simulink model "power_law_adapter"  (R2020b)
settings: Solver=FixedStepDiscrete  StartTime=0.0  StopTime=stopTime  FixedStep=2.0833333333333333e-05  RelTol=1e-3
undefined symbols (not defined in the file or in its folder): alpha1, alpha2, fast_coeffs, slow_coeffs
settings Model: Creator=Ross  LastModifiedBy=tyler
settings DataIOCC: SaveOutput=off  SaveTime=off  ReturnWorkspaceOutputs=off
settings OptimizationCC: BlockReduction=off  ConditionallyExecuteInputs=off  DefaultParameterBehavior=Inlined
settings DebuggingCC: ReadBeforeWriteMsg=DisableAll  WriteAfterWriteMsg=DisableAll  WriteAfterReadMsg=DisableAll  AlgebraicLoopMsg=error  MultiTaskDSMMsg=none  SingleTaskRateTransMsg=error  PregeneratedLibrarySubsystemCodeDiagnostic=none  ArithmeticOperatorsInVariantConditions=warning
settings HardwareCC: ProdBitPerPointer=32  ProdBitPerSizeT=32  ProdBitPerPtrDiffT=32  ProdLargestAtomicFloat=None  ProdIntDivRoundTo=Undefined  ProdEndianess=Unspecified  ProdWordSize=32  ProdHWDeviceType=ASIC/FPGA->ASIC/FPGA  TargetBitPerPointer=64  TargetBitPerSizeT=64  TargetBitPerPtrDiffT=64  TargetLongLongMode=on  TargetIntDivRoundTo=Zero  TargetEndianess=LittleEndian  TargetWordSize=64  TargetHWDeviceType=Custom Processor->MATLAB Host Computer  ProdEqTarget=off
settings ModelReferenceCC: UpdateModelReferenceTargets=IfOutOfDate
settings SFSimCC: SFSimEcho=off  SimUseLocalCustomCode=off  CustomCodeUndefinedFunction=UseInterfaceOnly
settings RTWCC: RTWUseLocalCustomCode=off

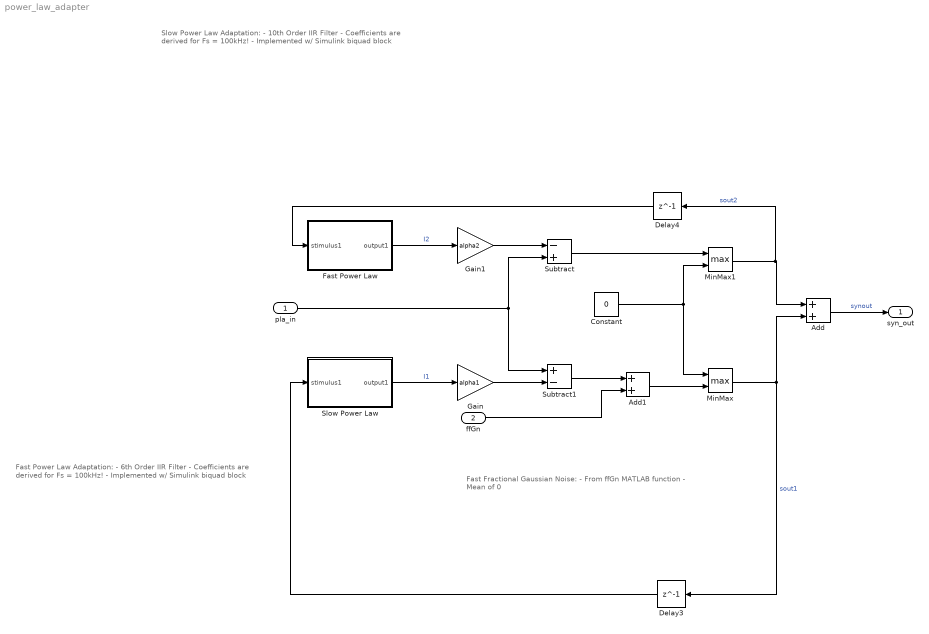
== system power_law_adapter ==
  note: Slow Power Law Adaptation:
      |
      | - 10th Order IIR Filter
      |
      | - Coefficients are derived for Fs = 100kHz!
      |
      | - Implemented w/ Simulink biquad block
  note: Fast Power Law Adaptation:
      |
      | - 6th Order IIR Filter
      |
      | - Coefficients are derived for Fs = 100kHz!
      |
      | - Implemented w/ Simulink biquad block
  note: Fast Fractional Gaussian Noise:
      |
      | - From ffGn MATLAB function
      |
      | - Mean of 0
  pla_in : Inport  OutDataTypeStr=single  PortDimensions=1  SampleTime=[2.0833333333333333e-05,0]
  ffGn : Inport  Port=2  OutDataTypeStr=single  PortDimensions=[1 1]  SampleTime=[2.0833333333333333e-05,0]
  Add : Sum
  Add1 : Sum
  Constant : Constant  Value=0  OutDataTypeStr=single  SampleTime=-1
  Delay3 : Delay  DelayLength=1
  Delay4 : Delay  DelayLength=1
  Fast Power Law : Subsystem
  Gain : Gain  Gain=alpha1  ParamDataTypeStr=single  OutDataTypeStr=single
  Gain1 : Gain  Gain=alpha2  ParamDataTypeStr=single  OutDataTypeStr=single
  MinMax : MinMax  Function=max  Inputs=2
  MinMax1 : MinMax  Function=max  Inputs=2
  Slow Power Law : Subsystem
  Subtract : Sum  Inputs=-+
  Subtract1 : Sum  Inputs=+-
  syn_out : Outport  OutDataTypeStr=single  PortDimensions=1  SampleTime=[2.0833333333333333e-05,0]
  wires:
  Subtract/1 -> MinMax1/1
  MinMax1/1 -> Delay4/1, Add/1  "sout2"
  Gain/1 -> Subtract1/2
  Fast Power Law/1(output1) -> Gain1/1  "I2"
  Gain1/1 -> Subtract/1
  Add1/1 -> MinMax/2
  Add/1 -> syn_out/1  "synout"
  Subtract1/1 -> Add1/1
  Constant/1 -> MinMax/1, MinMax1/2
  Slow Power Law/1(output1) -> Gain/1  "I1"
  MinMax/1 -> Delay3/1, Add/2  "sout1"
  Delay3/1 -> Slow Power Law/1(stimulus1)
  Delay4/1 -> Fast Power Law/1(stimulus1)
  ffGn/1 -> Add1/2
  pla_in/1 -> Subtract1/1, Subtract/2

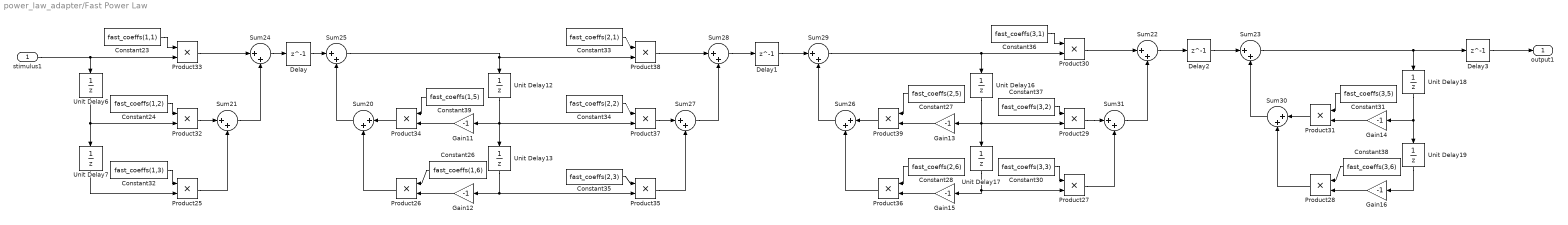
== system power_law_adapter/Fast Power Law ==
  stimulus1 : Inport
  Constant23 : Constant  Value=fast_coeffs(1,1)  OutDataTypeStr=single  SampleTime=-1
  Constant24 : Constant  Value=fast_coeffs(1,2)  OutDataTypeStr=single  SampleTime=-1
  Constant26 : Constant  Value=fast_coeffs(1,6)  OutDataTypeStr=single  SampleTime=-1
  Constant27 : Constant  Value=fast_coeffs(2,5)  OutDataTypeStr=single  SampleTime=-1
  Constant28 : Constant  Value=fast_coeffs(2,6)  OutDataTypeStr=single  SampleTime=-1
  Constant30 : Constant  Value=fast_coeffs(3,3)  OutDataTypeStr=single  SampleTime=-1
  Constant31 : Constant  Value=fast_coeffs(3,5)  OutDataTypeStr=single  SampleTime=-1
  Constant32 : Constant  Value=fast_coeffs(1,3)  OutDataTypeStr=single  SampleTime=-1
  Constant33 : Constant  Value=fast_coeffs(2,1)  OutDataTypeStr=single  SampleTime=-1
  Constant34 : Constant  Value=fast_coeffs(2,2)  OutDataTypeStr=single  SampleTime=-1
  Constant35 : Constant  Value=fast_coeffs(2,3)  OutDataTypeStr=single  SampleTime=-1
  Constant36 : Constant  Value=fast_coeffs(3,1)  OutDataTypeStr=single  SampleTime=-1
  Constant37 : Constant  Value=fast_coeffs(3,2)  OutDataTypeStr=single  SampleTime=-1
  Constant38 : Constant  Value=fast_coeffs(3,6)  OutDataTypeStr=single  SampleTime=-1
  Constant39 : Constant  Value=fast_coeffs(1,5)  OutDataTypeStr=single  SampleTime=-1
  Delay{,1..3} (4 alike) : Delay  DelayLength=1
  Gain{11..16} (6 alike) : Gain  Gain=-1
  Product{25..39} (15 alike) : Product
  Sum{20..31} (12 alike) : Sum  Inputs=|++
  Unit Delay{6..7,12..13,16..19} (8 alike) : UnitDelay  SampleTime=-1  HasFrameUpgradeWarning=on
  output1 : Outport  VectorParamsAs1DForOutWhenUnconnected=off
  wires:
  Product28/1 -> Sum30/2
  Gain12/1 -> Product26/2
  Constant28/1 -> Product36/1
  Constant31/1 -> Product31/1
  Constant38/1 -> Product28/1
  Constant37/1 -> Product29/1
  Constant30/1 -> Product27/1
  Product29/1 -> Sum31/1
  Unit Delay18/1 -> Unit Delay19/1, Gain14/1
  Constant36/1 -> Product30/1
  Sum31/1 -> Sum22/2
  Gain14/1 -> Product31/2
  Product35/1 -> Sum27/2
  Constant24/1 -> Product32/1
  Product36/1 -> Sum26/2
  Product39/1 -> Sum26/1
  Sum30/1 -> Sum23/2
  Constant35/1 -> Product35/1
  Product25/1 -> Sum21/2
  Constant23/1 -> Product33/1
  Product30/1 -> Sum22/1
  Unit Delay13/1 -> Product35/2, Gain12/1
  Constant33/1 -> Product38/1
  Unit Delay7/1 -> Product25/2
  Unit Delay17/1 -> Product27/2, Gain15/1
  Sum29/1 -> Product30/2, Unit Delay16/1
  Sum20/1 -> Sum25/2
  Sum26/1 -> Sum29/2
  Constant27/1 -> Product39/1
  Gain16/1 -> Product28/2
  Gain15/1 -> Product36/2
  Product32/1 -> Sum21/1
  Product31/1 -> Sum30/1
  Gain13/1 -> Product39/2
  Sum27/1 -> Sum28/2
  Constant34/1 -> Product37/1
  Product33/1 -> Sum24/1
  Product27/1 -> Sum31/2
  Unit Delay12/1 -> Product37/2, Unit Delay13/1, Gain11/1
  Sum25/1 -> Product38/2, Unit Delay12/1
  Unit Delay19/1 -> Gain16/1
  Product34/1 -> Sum20/1
  Gain11/1 -> Product34/2
  Sum24/1 -> Delay/1
  Constant32/1 -> Product25/1
  Product38/1 -> Sum28/1
  Product37/1 -> Sum27/1
  Sum21/1 -> Sum24/2
  Constant39/1 -> Product34/1
  Unit Delay6/1 -> Unit Delay7/1, Product32/2
  Unit Delay16/1 -> Product29/2, Unit Delay17/1, Gain13/1
  Constant26/1 -> Product26/1
  Product26/1 -> Sum20/2
  stimulus1/1 -> Product33/2, Unit Delay6/1
  Sum23/1 -> Delay3/1, Unit Delay18/1
  Delay/1 -> Sum25/1
  Sum28/1 -> Delay1/1
  Delay1/1 -> Sum29/1
  Delay2/1 -> Sum23/1
  Sum22/1 -> Delay2/1
  Delay3/1 -> output1/1

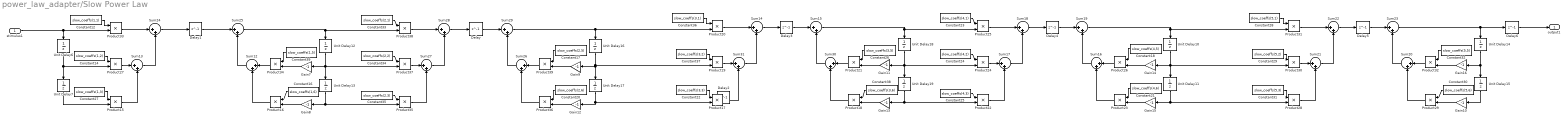
== system power_law_adapter/Slow Power Law ==
  stimulus1 : Inport
  Constant12 : Constant  Value=slow_coeffs(1,1)  OutDataTypeStr=single  SampleTime=-1
  Constant14 : Constant  Value=slow_coeffs(1,2)  OutDataTypeStr=single  SampleTime=-1
  Constant16 : Constant  Value=slow_coeffs(1,6)  OutDataTypeStr=single  SampleTime=-1
  Constant17 : Constant  Value=slow_coeffs(2,5)  OutDataTypeStr=single  SampleTime=-1
  Constant18 : Constant  Value=slow_coeffs(4,5)  OutDataTypeStr=single  SampleTime=-1
  Constant20 : Constant  Value=slow_coeffs(2,6)  OutDataTypeStr=single  SampleTime=-1
  Constant21 : Constant  Value=slow_coeffs(4,6)  OutDataTypeStr=single  SampleTime=-1
  Constant22 : Constant  Value=slow_coeffs(3,3)  OutDataTypeStr=single  SampleTime=-1
  Constant23 : Constant  Value=slow_coeffs(4,1)  OutDataTypeStr=single  SampleTime=-1
  Constant24 : Constant  Value=slow_coeffs(4,2)  OutDataTypeStr=single  SampleTime=-1
  Constant25 : Constant  Value=slow_coeffs(4,3)  OutDataTypeStr=single  SampleTime=-1
  Constant26 : Constant  Value=slow_coeffs(3,5)  OutDataTypeStr=single  SampleTime=-1
  Constant27 : Constant  Value=slow_coeffs(1,3)  OutDataTypeStr=single  SampleTime=-1
  Constant28 : Constant  Value=slow_coeffs(5,1)  OutDataTypeStr=single  SampleTime=-1
  Constant29 : Constant  Value=slow_coeffs(5,2)  OutDataTypeStr=single  SampleTime=-1
  Constant30 : Constant  Value=slow_coeffs(5,6)  OutDataTypeStr=single  SampleTime=-1
  Constant31 : Constant  Value=slow_coeffs(5,3)  OutDataTypeStr=single  SampleTime=-1
  Constant32 : Constant  Value=slow_coeffs(5,5)  OutDataTypeStr=single  SampleTime=-1
  Constant33 : Constant  Value=slow_coeffs(2,1)  OutDataTypeStr=single  SampleTime=-1
  Constant34 : Constant  Value=slow_coeffs(2,2)  OutDataTypeStr=single  SampleTime=-1
  Constant35 : Constant  Value=slow_coeffs(2,3)  OutDataTypeStr=single  SampleTime=-1
  Constant36 : Constant  Value=slow_coeffs(3,1)  OutDataTypeStr=single  SampleTime=-1
  Constant37 : Constant  Value=slow_coeffs(3,2)  OutDataTypeStr=single  SampleTime=-1
  Constant38 : Constant  Value=slow_coeffs(3,6)  OutDataTypeStr=single  SampleTime=-1
  Constant39 : Constant  Value=slow_coeffs(1,5)  OutDataTypeStr=single  SampleTime=-1
  Delay{,1..6} (7 alike) : Delay  DelayLength=1
  Gain{7..16} (10 alike) : Gain  Gain=-1
  Product{15..39} (25 alike) : Product
  Sum{12..31} (20 alike) : Sum  Inputs=|++
  Unit Delay{6..7,10..19} (12 alike) : UnitDelay  SampleTime=-1  HasFrameUpgradeWarning=on
  output1 : Outport  VectorParamsAs1DForOutWhenUnconnected=off
  wires:
  Gain11/1 -> Product21/2
  Sum17/1 -> Sum18/2
  Sum31/1 -> Sum14/2
  Sum16/1 -> Sum19/2
  Sum15/1 -> Product25/2, Unit Delay18/1
  Product21/1 -> Sum30/1
  Constant36/1 -> Product20/1
  Constant21/1 -> Product23/1
  Gain14/1 -> Product26/2
  Unit Delay18/1 -> Product24/2, Unit Delay19/1, Gain11/1
  Product24/1 -> Sum17/1
  Unit Delay11/1 -> Product28/2, Gain15/1
  Unit Delay10/1 -> Product30/2, Unit Delay11/1, Gain14/1
  Product20/1 -> Sum14/1
  Product19/1 -> Sum31/1
  Constant38/1 -> Product18/1
  Sum19/1 -> Product31/2, Unit Delay10/1
  Product25/1 -> Sum18/1
  Unit Delay19/1 -> Product22/2, Gain13/1
  Constant18/1 -> Product26/1
  Sum30/1 -> Sum15/2
  Constant26/1 -> Product21/1
  Product18/1 -> Sum30/2
  Constant22/1 -> Product17/1
  Product23/1 -> Sum16/2
  Constant37/1 -> Product19/1
  Constant25/1 -> Product22/1
  Constant23/1 -> Product25/1
  stimulus1/1 -> Product33/2, Unit Delay6/1
  Sum13/1 -> Sum24/2
  Constant30/1 -> Product29/1
  Gain7/1 -> Product34/2
  Sum27/1 -> Sum28/2
  Product22/1 -> Sum17/2
  Constant20/1 -> Product36/1
  Gain8/1 -> Product16/2
  Product34/1 -> Sum12/1
  Gain12/1 -> Product36/2
  Gain13/1 -> Product18/2
  Sum25/1 -> Product38/2, Unit Delay12/1
  Constant24/1 -> Product24/1
  Product33/1 -> Sum24/1
  Product37/1 -> Sum27/1
  Constant16/1 -> Product16/1
  Unit Delay16/1 -> Unit Delay17/1, Gain9/1, Product19/2
  Constant39/1 -> Product34/1
  Unit Delay17/1 -> Product17/2, Gain12/1
  Unit Delay7/1 -> Product15/2
  Product38/1 -> Sum28/1
  Unit Delay13/1 -> Product35/2, Gain8/1
  Constant12/1 -> Product33/1
  Product15/1 -> Sum13/2
  Constant33/1 -> Product38/1
  Gain15/1 -> Product23/2
  Product16/1 -> Sum12/2
  Constant35/1 -> Product35/1
  Sum12/1 -> Sum25/2
  Sum26/1 -> Sum29/2
  Constant17/1 -> Product39/1
  Product39/1 -> Sum26/1
  Product36/1 -> Sum26/2
  Product35/1 -> Sum27/2
  Constant27/1 -> Product15/1
  Constant32/1 -> Product32/1
  Sum20/1 -> Sum23/2
  Constant31/1 -> Product28/1
  Product29/1 -> Sum20/2
  Product28/1 -> Sum21/2
  Gain16/1 -> Product32/2
  Constant34/1 -> Product37/1
  Product32/1 -> Sum20/1
  Sum23/1 -> Delay6/1, Unit Delay14/1
  Gain10/1 -> Product29/2
  Product17/1 -> Sum31/2
  Unit Delay12/1 -> Product37/2, Unit Delay13/1, Gain7/1
  Constant29/1 -> Product30/1
  Sum29/1 -> Product20/2, Unit Delay16/1
  Constant28/1 -> Product31/1
  Sum21/1 -> Sum22/2
  Product30/1 -> Sum21/1
  Product27/1 -> Sum13/1
  Unit Delay14/1 -> Unit Delay15/1, Gain16/1
  Product26/1 -> Sum16/1
  Product31/1 -> Sum22/1
  Gain9/1 -> Product39/2
  Unit Delay15/1 -> Gain10/1
  Unit Delay6/1 -> Unit Delay7/1, Product27/2
  Constant14/1 -> Product27/1
  Sum28/1 -> Delay/1
  Delay/1 -> Sum29/1
  Delay1/1 -> Sum25/1
  Sum24/1 -> Delay1/1
  Sum14/1 -> Delay3/1
  Delay3/1 -> Sum15/1
  Sum18/1 -> Delay4/1
  Delay4/1 -> Sum19/1
  Sum22/1 -> Delay5/1
  Delay5/1 -> Sum23/1
  Delay6/1 -> output1/1
